simulink model "InctanceConfig"  (R2023a)
settings: Solver=VariableStepAuto  StartTime=0.0  StopTime=10.0  RelTol=1e-3
undefined symbols (not defined in the file or in its folder): gray
libraries: sim3dcameralib x3, sim3dautolib x2, sim3dlib x1
settings Model: Creator=Franz  LastModifiedBy=Franz

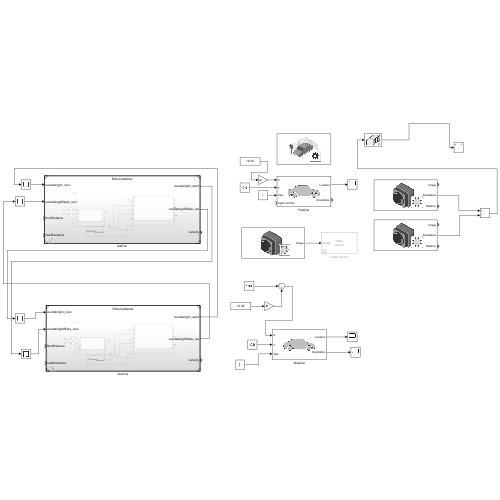
[thumbnail: Simulink's stored preview of the top-level diagram]
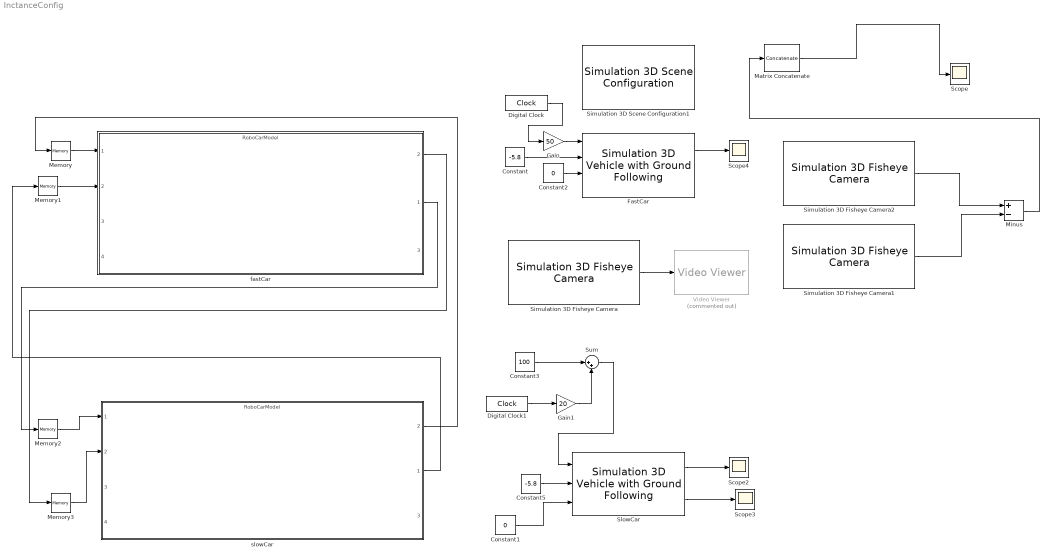
== system InctanceConfig ==
  Constant : Constant  Value=-5.8
  Constant1 : Constant  Value=0
  Constant2 : Constant  Value=0
  Constant3 : Constant  Value=100
  Constant5 : Constant  Value=-5.8
  Digital Clock : DigitalClock  SampleTime=0.01
  Digital Clock1 : DigitalClock  SampleTime=0.01
  FastCar : sim3dautolib/Simulation 3D Vehicle with Ground Following  Priority=-1  PassVehMesh=Muscle car  MeshPath=/MathWorksAutomotiveContent/Vehicles/Muscle/Meshes/SK_MuscleCar.SK_MuscleCar  TrackWidth=1.9  WheelBase=3  WheelRadius=0.35  VehColor=Red  InitialPos=[35,-5.8,0]  InitialRot=[0, 0, 0]  ActorName=FastCar  SampleTime=-1  ActorType=SimulinkVehicle  ID=C  aMode=3  ActorTag=FastCar  CoordinateScheme=ISO  VehLightsControl=on  HeadlightColor=[ 1, 1, 1 ]  HighBeamIntensity=100000  LowBeamIntensity=60000  HighBeamConeAngle=70  LowBeamConeAngle=70  LeftHeadlightOrientation=[ 0, 0 ]  RightHeadlightOrientation=[ 0, 0 ]  BrakelightIntensity=500  ReverselightIntensity=500  SignallightIntensity=500  SignallightPeriod=1  SignalPulseWidth=50  TransformOutportEnabled=on
      settings: LibrarySourceBlock=drivingsim3d/Simulation 3D Vehicle with Ground Following
  Gain : Gain  Gain=50
  Gain1 : Gain  Gain=20
  Matrix Concatenate : Concatenate  NumInputs=1  Mode=Multidimensional array  ConcatenateDimension=2
  Memory{,1..3} (4 alike) : Memory
  Minus : Sum  Inputs=+-
  Scope{,2..4} (4 alike) : Scope
  Simulation 3D Fisheye Camera : sim3dcameralib/Simulation 3D Fisheye Camera  Priority=1  sensorTag=Sim3dSensor1  sensorId=1  sensorName=Sim3dSensor1  vehTagList={'FastCar';'FastCarActor';'Scene Origin';'SlowCar'}  vehTag=FastCar  mountLoc=Roof center  offsetFlag=off  tmountOffset=[0, 0, 0]  extTmount=off  rmountOffset=[0, 0, 0]  extRmount=off  OpticalCenter=[640, 360]  ImageSize=[720, 1280]  RadialDistortion=[320, 0, 0, 0]  StretchMatrix=[1, 0; 0, 1]  TransformOutportEnabled=off  SampleTime=-1  mountPoint=[-0.25 0 1.57000005245209]  mountOrientation=[0 0 0]  aMode=3  ID=1
      settings: LibrarySourceBlock=drivingsim3d/Simulation 3D Fisheye Camera
  Simulation 3D Fisheye Camera1 : sim3dcameralib/Simulation 3D Fisheye Camera  Priority=1  sensorTag=Sim3dSensor6  sensorId=6  sensorName=Sim3dSensor6  vehTagList={'FastCar';'Scene Origin';'SlowCar'}  vehTag=FastCar  mountLoc=Origin  offsetFlag=off  tmountOffset=[0, 0, 0]  extTmount=off  rmountOffset=[0, 0, 0]  extRmount=off  OpticalCenter=[640, 360]  ImageSize=[720, 1280]  RadialDistortion=[320, 0, 0, 0]  StretchMatrix=[1, 0; 0, 1]  TransformOutportEnabled=on  SampleTime=-1  mountPoint=[0 0 0]  mountOrientation=[0 0 0]  aMode=3  ID=6
      settings: LibrarySourceBlock=drivingsim3d/Simulation 3D Fisheye Camera
  Simulation 3D Fisheye Camera2 : sim3dcameralib/Simulation 3D Fisheye Camera  Priority=1  sensorTag=Sim3dSensor7  sensorId=7  sensorName=Sim3dSensor7  vehTagList={'FastCar';'Scene Origin';'SlowCar'}  vehTag=SlowCar  mountLoc=Origin  offsetFlag=off  tmountOffset=[0, 0, 0]  extTmount=off  rmountOffset=[0, 0, 0]  extRmount=off  OpticalCenter=[640, 360]  ImageSize=[720, 1280]  RadialDistortion=[320, 0, 0, 0]  StretchMatrix=[1, 0; 0, 1]  TransformOutportEnabled=on  SampleTime=-1  mountPoint=[0 0 0]  mountOrientation=[0 0 0]  aMode=3  ID=7
      settings: LibrarySourceBlock=drivingsim3d/Simulation 3D Fisheye Camera
  Simulation 3D Scene Configuration1 : sim3dlib/Simulation 3D Scene Configuration  Priority=0  ProjectFormat=Default Scenes  SceneDesc=Double lane change  ProjectName=D:\Program Files\MATLAB\R2023a\toolbox\shared\sim3d_projects\automotive_project\UE4\WindowsNoEditor\VehicleSimulation.exe  ScenePath=/Game/Maps/HwStrght  EnableOpenDRIVE=off  vehTagList={'FastCar';'Scene Origin';'SlowCar'}  vehTag=FastCar  OpVisEn=off  Ts=1/60  EnableWindow=on  EnableRemoteAccess=off  EnableWeather=off  SunAltitude=40.0  SunAzimuth=90  clouds=10  wind=1  fog=0  rain=0  EnableGeospatial=off  OriginHeight=200  OriginLatitude=40.744652  OriginLongitude=-73.988864  MapStyle=Aerial  AdditionalAssetIDs=[]  UseAdvancedSunSky=off  SolarTime=11  TimeZone=-5  Day=21  Month=9  Year=2022  UseDaylightSavingTime=on  DSTStartDay=10  DSTStartMonth=3  DSTEndDay=3  DSTEndMonth=11  DSTSwitchHour=2  sensorTag=MainCamera2  sensorId=2  sensorName=MainCamera2  mountLoc=Origin  offsetFlag=off  tmountOffset=[0, 0, 0]  rmountOffset=[0, 0, 0]  HorizontalResolution=1280  VerticalResolution=720  HorizontalFOV=60  mountPoint=[0 0 0]  mountOrientation=[0 0 0]  aMode=3  ID=2  GeoTrigger=Inactive
      settings: LibrarySourceBlock=drivingsim3d/Simulation 3D Scene Configuration
  SlowCar : sim3dautolib/Simulation 3D Vehicle with Ground Following  Priority=-1  PassVehMesh=Muscle car  MeshPath=/MathWorksAutomotiveContent/Vehicles/Muscle/Meshes/SK_MuscleCar.SK_MuscleCar  TrackWidth=1.9  WheelBase=3  WheelRadius=0.35  VehColor=Green  InitialPos=[0, 0, 0]  InitialRot=[0, 0, 0]  ActorName=SlowCar  SampleTime=-1  ActorType=SimulinkVehicle  ID=C  aMode=3  ActorTag=SlowCar  CoordinateScheme=ISO  VehLightsControl=off  HeadlightColor=[ 1, 1, 1 ]  HighBeamIntensity=100000  LowBeamIntensity=60000  HighBeamConeAngle=70  LowBeamConeAngle=70  LeftHeadlightOrientation=[ 0, 0 ]  RightHeadlightOrientation=[ 0, 0 ]  BrakelightIntensity=500  ReverselightIntensity=500  SignallightIntensity=500  SignallightPeriod=1  SignalPulseWidth=50  TransformOutportEnabled=on
      settings: LibrarySourceBlock=drivingsim3d/Simulation 3D Vehicle with Ground Following
  Sum : Sum  Inputs=|++
  Video Viewer : VideoViewer  Commented=on  colormapValue=gray(256)  FigPos=[399 900 1271 692]
  fastCar : ModelReference  ModelNameDialog=RoboCarModel.slx  SimulationMode=Normal  ModelReferenceVersion=1.94
      settings: PortSchema="{\"entries\":[{\"content\":{\"sides\":[{\"content\":{\"connectorIds\":[\"In1\",\"In2\",\"In3\",\"In4\"]},\"type\":\"ConnectorPlacement.EquallySpacedRectSide\",\"uuid\":\"95733cf0-032d-453a-9995-7e8d3e1a24c3\"},{\"content\":{\"connectorIds\":[\"Out2\",\"Out1\",\"Out3\"],\"side\":\"RIGHT\"},\"type\":\"ConnectorPlacement.EquallySpacedRectSide\",\"uuid\":\"8d40af39-e74b-4bad-b693-9b5567a60d93\"},{\"content\":{\"side\":\"TOP\"},\"type\":\"ConnectorPlacement.EquallySpacedRectSide\",\"uuid\":\"43bbd94f-fc32-448c-b6cd-ad2d068142f7\"}]},\"type\":\"ConnectorPlacement.EquallySpacedConnector\",\"uuid\":\"f2b8ce5d-c214-4fd8-985d-570b817192f6\"}],\"packageUris\":[\"http://schema.mathworks.com/mf0/Connector/R2020b\"],\"version\":\"1.0\"}"
  slowCar : ModelReference  ModelNameDialog=RoboCarModel.slx  SimulationMode=Normal  ModelReferenceVersion=1.94
      settings: PortSchema="{\"entries\":[{\"content\":{\"sides\":[{\"content\":{\"connectorIds\":[\"In1\",\"In2\",\"In3\",\"In4\"]},\"type\":\"ConnectorPlacement.EquallySpacedRectSide\",\"uuid\":\"95733cf0-032d-453a-9995-7e8d3e1a24c3\"},{\"content\":{\"connectorIds\":[\"Out2\",\"Out1\",\"Out3\"],\"side\":\"RIGHT\"},\"type\":\"ConnectorPlacement.EquallySpacedRectSide\",\"uuid\":\"8d40af39-e74b-4bad-b693-9b5567a60d93\"},{\"content\":{\"side\":\"TOP\"},\"type\":\"ConnectorPlacement.EquallySpacedRectSide\",\"uuid\":\"43bbd94f-fc32-448c-b6cd-ad2d068142f7\"}]},\"type\":\"ConnectorPlacement.EquallySpacedConnector\",\"uuid\":\"f2b8ce5d-c214-4fd8-985d-570b817192f6\"}],\"packageUris\":[\"http://schema.mathworks.com/mf0/Connector/R2020b\"],\"version\":\"1.0\"}"
  wires:
  fastCar/1 -> Memory2/1
  slowCar/2 -> Memory/1
  slowCar/1 -> Memory1/1
  fastCar/2 -> Memory3/1
  Simulation 3D Fisheye Camera/1 -> Video Viewer/1
  Memory/1 -> fastCar/1
  Memory1/1 -> fastCar/2
  Memory2/1 -> slowCar/1
  Memory3/1 -> slowCar/2
  SlowCar/1 -> Scope2/1
  SlowCar/2 -> Scope3/1
  Constant5/1 -> SlowCar/2
  Gain/1 -> FastCar/1
  Digital Clock/1 -> Gain/1
  Constant/1 -> FastCar/2
  Constant2/1 -> FastCar/3
  Constant1/1 -> SlowCar/3
  Constant3/1 -> Sum/1
  Digital Clock1/1 -> Gain1/1
  Gain1/1 -> Sum/2
  Sum/1 -> SlowCar/1
  FastCar/1 -> Scope4/1
  Simulation 3D Fisheye Camera1/2 -> Minus/2
  Simulation 3D Fisheye Camera2/2 -> Minus/1
  Matrix Concatenate/1 -> Scope/1
  Minus/1 -> Matrix Concatenate/1
